simulink model "A_3_5"  (R2025b)
settings: Solver=VariableStepAuto  StartTime=0.0  StopTime=10.0  RelTol=1e-3
settings Model: Creator=alaraerol  LastModifiedBy=alaraerol

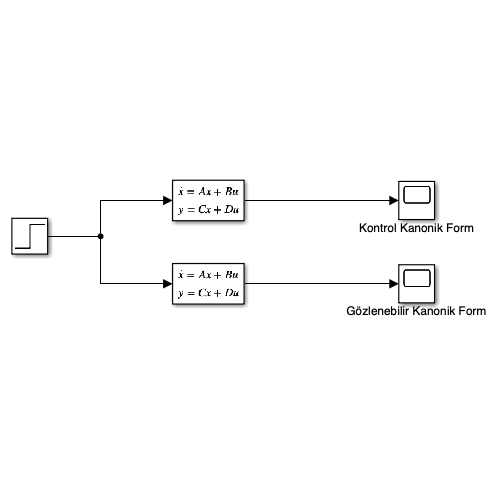
[thumbnail: Simulink's stored preview of the top-level diagram]
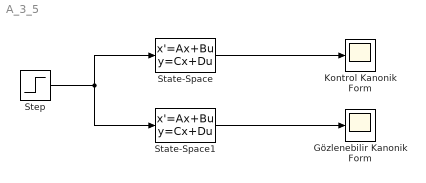
== system A_3_5 ==
  Gözlenebilir Kanonik Form : Scope
  Kontrol Kanonik Form : Scope
  State-Space : StateSpace  A=[0 1; -555.56 -15]  B=[0; 1]  C=[555.56 0]  D=0  InitialCondition=0
  State-Space1 : StateSpace  A=[0 -555.56;1 -15]  B=[555.56; 0]  C=[0 1]  D=0  InitialCondition=0
  Step : Step  SampleTime=0
  wires:
  State-Space/1 -> Kontrol Kanonik Form/1
  State-Space1/1 -> Gözlenebilir Kanonik Form/1
  Step/1 -> State-Space1/1, State-Space/1
